simulink library "PC_Simulator_Lib"  (Simulink 8.2)
settings: Solver=ode45  StartTime=0.0  StopTime=10.0  RelTol=1e-3
values from neighbouring files (symbols this model uses):
  data = [r1 r2 r3 r4 L1 L2 L3 L4]    [strasse_Bedatung_HNI_ITI.m]
  distSameLane = 60    [InitialisationsEnv.m]
  eng_speed = [0 60 120 180 240 300 360 420 480 540 600 660 ... (101 elements, 1x101)]    [engine_table.mat]    (also in motor_parameter_calc.m = omega)
  Heading_init = 0    [Start.m]
  inertiaLateral = 25*(radiusWheel)^2    (= 4.129024)    [Start.m]
  laneWidth = 3.6    [InitialisationsEnv.m]    (also in strasse_Bedatung_HNI_ITI.m)
  omega_engine = [0.000000 150.000000 500.000000 1000.000000 1500.000000 2000.000000 2500.000000 3000.000000 3500.000000 4000.000000 4500.000000 5000.000000 5500.000000 6000.000000]    [friction_tables.m]
  omega_max = 6000    [engine_table.mat]    (also in motor_parameter_calc.m)
  omega_wheel = [0 20 40 60 80 100 122 143.7 164]    [friction_tables.m]
  para_Fellow_8_Points = ADAS.Fellow_8_Points    [ADAS_parameters.m]
  position_start_x = [x1 x2 x3 x4 x5 x6 x7]    [strasse_Bedatung_HNI_ITI.m]
  position_start_y = [y1 y2 y3 y4 y5 y6 y7]    [strasse_Bedatung_HNI_ITI.m]
  rad3rdLine = 57.2    [InitialisationsEnv.m]    (also in strasse_Bedatung_HNI_ITI.m)
  radiusWheel = 16*2.54/100    (= 0.4064)    [Start.m]
  s_values = [S1 S2 S3 S4 S5 S6 S7]    [strasse_Bedatung_HNI_ITI.m]
  segmentLimits = [segment1EndThirdLine                   segment2EndThirdLine                   segment3EndThirdLine                   segment4EndThirdLine                   segment5EndThirdLine                   segment6EndThirdLine                   segment7EndThirdLine                   segment8EndThirdLine                   ]    [InitialisationsEnv.m]    (also in strasse_Bedatung_HNI_ITI.m)
  setPosT = [-1.8 -5.4 -1.8 -5.4 -1.8 -5.4 -1.8 -5.4 -1.8 -5.4]    [InitialisationsEnv.m]
  torque = [297.089227105 300.997600937 304.800343044 308.497453426 312.088932082 315.574779014 318.95499422 322.229577701 325.398529457 328.461849487 331.419537793 334.271594373 ... (101 elements, 1x101)]    [engine_table.mat]    (also in motor_parameter_calc.m = g)
  Torque_lost = [0.000000 -8.777780 -15.000000 -26.800000 -29.600000 -32.700000 -35.900000 -39.300000 -42.800000 -46.500000 -50.300000 -54.300000 -58.500000 -62.800000 ]*0.6    [friction_tables.m]
  Torque_lost_wheel = [0.8 0.8 0.75 0.7 0.4 0.3 0.2 0.07 0.07]*0.2    [friction_tables.m]
  X_init = 0    [Start.m]
  Y_init = 1.8    [Start.m]
  Z_init = 0    [Start.m]
undefined symbols (not defined in the file or in its folder): Acc_Pedal, ADAS, Brake_Pedal, Joystick, Newton, Para, Raphson, Standard_Devices, Steering_Wheel_Angle, UDP_Protocol
libraries: simulink x43, rtwinlib x7, dspnetwork x2, simulink_extras x1, vrlib x1
(part 9 of 13)

== system PC_Simulator_Lib/Environment/Environment_Model/Traffic_Vehicle_Model1/Vehicle_Model_s ==
  note: Vehicle acceleration = 0.3 m/s2
  note: Actual S velocity [m/s]
  note: Desired S velocity [m/s]
  ResetSig[] : Inport
  VelSDesired[Km/h] : Inport  Port=2
  Integrate acceleration to speed : Integrator  ExternalReset=rising
  Integrate speed to position : Integrator  ExternalReset=rising  InitialCondition=Para.EN.InitCond.S01
  Proportional Gain : Gain  Gain=10
  "Reset s position " : Math  Operator=mod  SaturateOnIntegerOverflow=on
  Road max length[m] : Constant  Value=2159
  Sum : Sum  Inputs=|+-
  Traffic vehicle model s direction First order system : TransferFcn  Denominator=[1 2*pi/0.3 ]
  "Transforn from  Km/h to m/s " : Gain  Gain=1/3.6
  VelS[m/s] : Outport
  PosS[m] : Outport  Port=2
  wires:
  VelSDesired[Km/h]/1 -> "Transforn from  Km/h to m/s "/1
  Integrate speed to position/1 -> "Reset s position "/1
  Road max length[m]/1 -> "Reset s position "/2
  "Transforn from  Km/h to m/s "/1 -> Sum/1
  ResetSig[]/1 -> Integrate acceleration to speed/2, Integrate speed to position/2
  "Reset s position "/1 -> PosS[m]/1
  Traffic vehicle model s direction First order system/1 -> Integrate acceleration to speed/1
  Integrate acceleration to speed/1 -> Sum/2, Integrate speed to position/1, VelS[m/s]/1
  Proportional Gain/1 -> Traffic vehicle model s direction First order system/1
  Sum/1 -> Proportional Gain/1

== system PC_Simulator_Lib/Environment/Environment_Model/Traffic_Vehicle_Model11/Vehicle_Model_s ==
  note: Desired S velocity [m/s]
  note: Actual S velocity [m/s]
  note: Vehicle acceleration = 0.3 m/s2
  ResetSig[] : Inport
  VelSDesired[Km/h] : Inport  Port=2
  Integrate acceleration to speed : Integrator  ExternalReset=rising
  Integrate speed to position : Integrator  ExternalReset=rising  InitialCondition=Para.EN.InitCond.S10
  Proportional Gain : Gain  Gain=10
  "Reset s position " : Math  Operator=mod  SaturateOnIntegerOverflow=on
  Road max length[m] : Constant  Value=2159
  Sum : Sum  Inputs=|+-
  Traffic vehicle model s direction First order system : TransferFcn  Denominator=[1 2*pi/0.3 ]
  "Transforn from  Km/h to m/s " : Gain  Gain=1/3.6
  VelS[m/s] : Outport
  PosS[m] : Outport  Port=2
  wires:
  Proportional Gain/1 -> Traffic vehicle model s direction First order system/1
  Sum/1 -> Proportional Gain/1
  Integrate acceleration to speed/1 -> VelS[m/s]/1, Integrate speed to position/1, Sum/2
  Traffic vehicle model s direction First order system/1 -> Integrate acceleration to speed/1
  "Reset s position "/1 -> PosS[m]/1
  ResetSig[]/1 -> Integrate speed to position/2, Integrate acceleration to speed/2
  "Transforn from  Km/h to m/s "/1 -> Sum/1
  Road max length[m]/1 -> "Reset s position "/2
  Integrate speed to position/1 -> "Reset s position "/1
  VelSDesired[Km/h]/1 -> "Transforn from  Km/h to m/s "/1

== system PC_Simulator_Lib/Environment/Environment_Model/Traffic_Vehicle_Model11/Vehicle_Model_t ==
  ResetSig[] : Inport
  PosTDesired[m] : Inport  Port=2
  Controller : Subsystem
  Integrator : Integrator  ExternalReset=rising  InitialCondition=-9
  Simple_vehicle_model_lateral : TransferFcn  Denominator=[0.2 1]
  Sum : Sum  Inputs=|+-
  PosT[m] : Outport
  wires:
  Sum/1 -> Controller/2(t_diff)
  Controller/1(v_ref) -> Simple_vehicle_model_lateral/1
  Integrator/1 -> PosT[m]/1, Sum/2
  Simple_vehicle_model_lateral/1 -> Integrator/1
  PosTDesired[m]/1 -> Sum/1
  ResetSig[]/1 -> Controller/1(ResetSig[]), Integrator/2

== system PC_Simulator_Lib/Environment/Environment_Model/Traffic_Vehicle_Model2/Vehicle_Model_s ==
  note: Vehicle acceleration = 0.3 m/s2
  note: Actual S velocity [m/s]
  note: Desired S velocity [m/s]
  ResetSig[] : Inport
  VelSDesired[Km/h] : Inport  Port=2
  Integrate acceleration to speed : Integrator  ExternalReset=rising
  Integrate speed to position : Integrator  ExternalReset=rising  InitialCondition=Para.EN.InitCond.S02
  Proportional Gain : Gain  Gain=10
  "Reset s position " : Math  Operator=mod  SaturateOnIntegerOverflow=on
  Road max length[m] : Constant  Value=2159
  Sum : Sum  Inputs=|+-
  Traffic vehicle model s direction First order system : TransferFcn  Denominator=[1 2*pi/0.3 ]
  "Transforn from  Km/h to m/s " : Gain  Gain=1/3.6
  VelS[m/s] : Outport
  PosS[m] : Outport  Port=2
  wires:
  VelSDesired[Km/h]/1 -> "Transforn from  Km/h to m/s "/1
  Integrate speed to position/1 -> "Reset s position "/1
  Road max length[m]/1 -> "Reset s position "/2
  "Transforn from  Km/h to m/s "/1 -> Sum/1
  ResetSig[]/1 -> Integrate acceleration to speed/2, Integrate speed to position/2
  "Reset s position "/1 -> PosS[m]/1
  Traffic vehicle model s direction First order system/1 -> Integrate acceleration to speed/1
  Integrate acceleration to speed/1 -> Sum/2, Integrate speed to position/1, VelS[m/s]/1
  Proportional Gain/1 -> Traffic vehicle model s direction First order system/1
  Sum/1 -> Proportional Gain/1

== system PC_Simulator_Lib/Environment/Environment_Model/Traffic_Vehicle_Model3/Vehicle_Model_s ==
  note: Vehicle acceleration = 0.3 m/s2
  note: Actual S velocity [m/s]
  note: Desired S velocity [m/s]
  ResetSig[] : Inport
  VelSDesired[Km/h] : Inport  Port=2
  Integrate acceleration to speed : Integrator  ExternalReset=rising
  Integrate speed to position : Integrator  ExternalReset=rising  InitialCondition=Para.EN.InitCond.S03
  Proportional Gain : Gain  Gain=10
  "Reset s position " : Math  Operator=mod  SaturateOnIntegerOverflow=on
  Road max length[m] : Constant  Value=2159
  Sum : Sum  Inputs=|+-
  Traffic vehicle model s direction First order system : TransferFcn  Denominator=[1 2*pi/0.3 ]
  "Transforn from  Km/h to m/s " : Gain  Gain=1/3.6
  VelS[m/s] : Outport
  PosS[m] : Outport  Port=2
  wires:
  VelSDesired[Km/h]/1 -> "Transforn from  Km/h to m/s "/1
  Integrate speed to position/1 -> "Reset s position "/1
  Road max length[m]/1 -> "Reset s position "/2
  "Transforn from  Km/h to m/s "/1 -> Sum/1
  ResetSig[]/1 -> Integrate acceleration to speed/2, Integrate speed to position/2
  "Reset s position "/1 -> PosS[m]/1
  Traffic vehicle model s direction First order system/1 -> Integrate acceleration to speed/1
  Integrate acceleration to speed/1 -> Sum/2, Integrate speed to position/1, VelS[m/s]/1
  Proportional Gain/1 -> Traffic vehicle model s direction First order system/1
  Sum/1 -> Proportional Gain/1

== system PC_Simulator_Lib/Environment/Environment_Model/Traffic_Vehicle_Model4/Vehicle_Model_s ==
  note: Vehicle acceleration = 0.3 m/s2
  note: Actual S velocity [m/s]
  note: Desired S velocity [m/s]
  ResetSig[] : Inport
  VelSDesired[Km/h] : Inport  Port=2
  Integrate acceleration to speed : Integrator  ExternalReset=rising
  Integrate speed to position : Integrator  ExternalReset=rising  InitialCondition=Para.EN.InitCond.S04
  Proportional Gain : Gain  Gain=10
  "Reset s position " : Math  Operator=mod  SaturateOnIntegerOverflow=on
  Road max length[m] : Constant  Value=2159
  Sum : Sum  Inputs=|+-
  Traffic vehicle model s direction First order system : TransferFcn  Denominator=[1 2*pi/0.3 ]
  "Transforn from  Km/h to m/s " : Gain  Gain=1/3.6
  VelS[m/s] : Outport
  PosS[m] : Outport  Port=2
  wires:
  VelSDesired[Km/h]/1 -> "Transforn from  Km/h to m/s "/1
  Integrate speed to position/1 -> "Reset s position "/1
  Road max length[m]/1 -> "Reset s position "/2
  "Transforn from  Km/h to m/s "/1 -> Sum/1
  ResetSig[]/1 -> Integrate acceleration to speed/2, Integrate speed to position/2
  "Reset s position "/1 -> PosS[m]/1
  Traffic vehicle model s direction First order system/1 -> Integrate acceleration to speed/1
  Integrate acceleration to speed/1 -> Sum/2, Integrate speed to position/1, VelS[m/s]/1
  Proportional Gain/1 -> Traffic vehicle model s direction First order system/1
  Sum/1 -> Proportional Gain/1

== system PC_Simulator_Lib/Environment/Environment_Model/Traffic_Vehicle_Model5/Vehicle_Model_s ==
  note: Vehicle acceleration = 0.3 m/s2
  note: Actual S velocity [m/s]
  note: Desired S velocity [m/s]
  ResetSig[] : Inport
  VelSDesired[Km/h] : Inport  Port=2
  Integrate acceleration to speed : Integrator  ExternalReset=rising
  Integrate speed to position : Integrator  ExternalReset=rising  InitialCondition=Para.EN.InitCond.S05
  Proportional Gain : Gain  Gain=10
  "Reset s position " : Math  Operator=mod  SaturateOnIntegerOverflow=on
  Road max length[m] : Constant  Value=2159
  Sum : Sum  Inputs=|+-
  Traffic vehicle model s direction First order system : TransferFcn  Denominator=[1 2*pi/0.3 ]
  "Transforn from  Km/h to m/s " : Gain  Gain=1/3.6
  VelS[m/s] : Outport
  PosS[m] : Outport  Port=2
  wires:
  VelSDesired[Km/h]/1 -> "Transforn from  Km/h to m/s "/1
  Integrate speed to position/1 -> "Reset s position "/1
  Road max length[m]/1 -> "Reset s position "/2
  "Transforn from  Km/h to m/s "/1 -> Sum/1
  ResetSig[]/1 -> Integrate acceleration to speed/2, Integrate speed to position/2
  "Reset s position "/1 -> PosS[m]/1
  Traffic vehicle model s direction First order system/1 -> Integrate acceleration to speed/1
  Integrate acceleration to speed/1 -> Sum/2, Integrate speed to position/1, VelS[m/s]/1
  Proportional Gain/1 -> Traffic vehicle model s direction First order system/1
  Sum/1 -> Proportional Gain/1

== system PC_Simulator_Lib/Environment/Environment_Model/Traffic_Vehicle_Model6/Vehicle_Model_s ==
  note: Vehicle acceleration = 0.3 m/s2
  note: Actual S velocity [m/s]
  note: Desired S velocity [m/s]
  ResetSig[] : Inport
  VelSDesired[Km/h] : Inport  Port=2
  Integrate acceleration to speed : Integrator  ExternalReset=rising
  Integrate speed to position : Integrator  ExternalReset=rising  InitialCondition=Para.EN.InitCond.S06
  Proportional Gain : Gain  Gain=10
  "Reset s position " : Math  Operator=mod  SaturateOnIntegerOverflow=on
  Road max length[m] : Constant  Value=2159
  Sum : Sum  Inputs=|+-
  Traffic vehicle model s direction First order system : TransferFcn  Denominator=[1 2*pi/0.3 ]
  "Transforn from  Km/h to m/s " : Gain  Gain=1/3.6
  VelS[m/s] : Outport
  PosS[m] : Outport  Port=2
  wires:
  VelSDesired[Km/h]/1 -> "Transforn from  Km/h to m/s "/1
  Integrate speed to position/1 -> "Reset s position "/1
  Road max length[m]/1 -> "Reset s position "/2
  "Transforn from  Km/h to m/s "/1 -> Sum/1
  ResetSig[]/1 -> Integrate acceleration to speed/2, Integrate speed to position/2
  "Reset s position "/1 -> PosS[m]/1
  Traffic vehicle model s direction First order system/1 -> Integrate acceleration to speed/1
  Integrate acceleration to speed/1 -> Sum/2, Integrate speed to position/1, VelS[m/s]/1
  Proportional Gain/1 -> Traffic vehicle model s direction First order system/1
  Sum/1 -> Proportional Gain/1

== system PC_Simulator_Lib/Environment/Environment_Model/Traffic_Vehicle_Model7/Vehicle_Model_s ==
  note: Vehicle acceleration = 0.3 m/s2
  note: Actual S velocity [m/s]
  note: Desired S velocity [m/s]
  ResetSig[] : Inport
  VelSDesired[Km/h] : Inport  Port=2
  Integrate acceleration to speed : Integrator  ExternalReset=rising
  Integrate speed to position : Integrator  ExternalReset=rising  InitialCondition=Para.EN.InitCond.S07
  Proportional Gain : Gain  Gain=10
  "Reset s position " : Math  Operator=mod  SaturateOnIntegerOverflow=on
  Road max length[m] : Constant  Value=2159
  Sum : Sum  Inputs=|+-
  Traffic vehicle model s direction First order system : TransferFcn  Denominator=[1 2*pi/0.3 ]
  "Transforn from  Km/h to m/s " : Gain  Gain=1/3.6
  VelS[m/s] : Outport
  PosS[m] : Outport  Port=2
  wires:
  VelSDesired[Km/h]/1 -> "Transforn from  Km/h to m/s "/1
  Integrate speed to position/1 -> "Reset s position "/1
  Road max length[m]/1 -> "Reset s position "/2
  "Transforn from  Km/h to m/s "/1 -> Sum/1
  ResetSig[]/1 -> Integrate acceleration to speed/2, Integrate speed to position/2
  "Reset s position "/1 -> PosS[m]/1
  Traffic vehicle model s direction First order system/1 -> Integrate acceleration to speed/1
  Integrate acceleration to speed/1 -> Sum/2, Integrate speed to position/1, VelS[m/s]/1
  Proportional Gain/1 -> Traffic vehicle model s direction First order system/1
  Sum/1 -> Proportional Gain/1

== system PC_Simulator_Lib/Environment/Environment_Model/Traffic_Vehicle_Model8/Vehicle_Model_s ==
  note: Vehicle acceleration = 0.3 m/s2
  note: Actual S velocity [m/s]
  note: Desired S velocity [m/s]
  ResetSig[] : Inport
  VelSDesired[Km/h] : Inport  Port=2
  Integrate acceleration to speed : Integrator  ExternalReset=rising
  Integrate speed to position : Integrator  ExternalReset=rising  InitialCondition=Para.EN.InitCond.S08
  Proportional Gain : Gain  Gain=10
  "Reset s position " : Math  Operator=mod  SaturateOnIntegerOverflow=on
  Road max length[m] : Constant  Value=2159
  Sum : Sum  Inputs=|+-
  Traffic vehicle model s direction First order system : TransferFcn  Denominator=[1 2*pi/0.3 ]
  "Transforn from  Km/h to m/s " : Gain  Gain=1/3.6
  VelS[m/s] : Outport
  PosS[m] : Outport  Port=2
  wires:
  VelSDesired[Km/h]/1 -> "Transforn from  Km/h to m/s "/1
  Integrate speed to position/1 -> "Reset s position "/1
  Road max length[m]/1 -> "Reset s position "/2
  "Transforn from  Km/h to m/s "/1 -> Sum/1
  ResetSig[]/1 -> Integrate acceleration to speed/2, Integrate speed to position/2
  "Reset s position "/1 -> PosS[m]/1
  Traffic vehicle model s direction First order system/1 -> Integrate acceleration to speed/1
  Integrate acceleration to speed/1 -> Sum/2, Integrate speed to position/1, VelS[m/s]/1
  Proportional Gain/1 -> Traffic vehicle model s direction First order system/1
  Sum/1 -> Proportional Gain/1

== system PC_Simulator_Lib/Environment/Environment_Model/Traffic_Vehicle_Model9/Vehicle_Model_s ==
  note: Vehicle acceleration = 0.3 m/s2
  note: Actual S velocity [m/s]
  note: Desired S velocity [m/s]
  ResetSig[] : Inport
  VelSDesired[Km/h] : Inport  Port=2
  Integrate acceleration to speed : Integrator  ExternalReset=rising
  Integrate speed to position : Integrator  ExternalReset=rising  InitialCondition=Para.EN.InitCond.S09
  Proportional Gain : Gain  Gain=10
  "Reset s position " : Math  Operator=mod  SaturateOnIntegerOverflow=on
  Road max length[m] : Constant  Value=2159
  Sum : Sum  Inputs=|+-
  Traffic vehicle model s direction First order system : TransferFcn  Denominator=[1 2*pi/0.3 ]
  "Transforn from  Km/h to m/s " : Gain  Gain=1/3.6
  VelS[m/s] : Outport
  PosS[m] : Outport  Port=2
  wires:
  VelSDesired[Km/h]/1 -> "Transforn from  Km/h to m/s "/1
  Integrate speed to position/1 -> "Reset s position "/1
  Road max length[m]/1 -> "Reset s position "/2
  "Transforn from  Km/h to m/s "/1 -> Sum/1
  ResetSig[]/1 -> Integrate acceleration to speed/2, Integrate speed to position/2
  "Reset s position "/1 -> PosS[m]/1
  Traffic vehicle model s direction First order system/1 -> Integrate acceleration to speed/1
  Integrate acceleration to speed/1 -> Sum/2, Integrate speed to position/1, VelS[m/s]/1
  Proportional Gain/1 -> Traffic vehicle model s direction First order system/1
  Sum/1 -> Proportional Gain/1

== system PC_Simulator_Lib/Vehicle dynamics/Vertical_Dyn./suspention_System/Rear_Right_Suspention ==
  note: Fs=f0s+KU
  note: Fs=K(Lf-(L0 - U))
  note: U
  note: Spring_intial_length+Spring_precompressed_length = Spring_Free_length
  note: Vertical_Velocity_Z_vehicle_corner_RR
  Vertical_Displacement_Z_vehicle_corner_RR : Inport
  Vertical_Displacement_Z0 : Inport  Port=2
  intial_force_form_mass_rr : Inport  Port=3
  Add1 : Sum  Inputs=+++
  Add2 : Sum  Inputs=+-
  Constant : Constant  Value=0
  Constant2 : Constant  Value=Para.VD.Spring_intial_length.v
  Gain : Gain  Gain=Para.VD.Spring_Stifness_Rear.v
  Gain2 : Gain  Gain=Para.VD.Damper_Damping_Constant_Rear.v
  Relational Operator : RelationalOperator  Operator=>  OutDataTypeStr=boolean  ZeroCross=off
  Relational Operator1 : RelationalOperator  Operator=<  OutDataTypeStr=boolean  ZeroCross=off
  Saturation : Saturate  UpperLimit=Para.VD.Spring_intial_length.v-Para.VD.Spring_Lower_limit.v  LowerLimit=Para.VD.Spring_intial_length.v-Para.VD.Spring_Upper_limit.v
  Subtract : Sum  Inputs=+-
  Subtract1 : Sum  Inputs=+-
  Subtract2 : Sum  Inputs=+-
  Switch : Switch
  Switch1 : Switch
  Transfer Fcn : TransferFcn  Numerator=[1 0]  Denominator=[0.001 1]
  vertical_dynamics_tire : Subsystem
  Force_Suspention_RR : Outport
  Hight_Reer_Right : Outport  Port=2
  Z1 : Outport  Port=3
  Z2actual : Outport  Port=4
  wires:
  Subtract2/1 -> Hight_Reer_Right/1
  Constant2/1 -> Subtract2/1
  Transfer Fcn/1 -> Subtract1/2
  Vertical_Displacement_Z_vehicle_corner_RR/1 -> Subtract/2, Transfer Fcn/1, Switch/3
  Subtract/1 -> Saturation/1, Relational Operator/1, Relational Operator1/1
  Saturation/1 -> Gain/1, Subtract2/2, Add2/2, Relational Operator/2, Relational Operator1/2
  Add1/1 -> Force_Suspention_RR/1, vertical_dynamics_tire/1(Force_Suspention)
  Gain2/1 -> Add1/2
  Subtract1/1 -> Gain2/1
  Gain/1 -> Add1/1
  vertical_dynamics_tire/1(Vertical_Displacement_Z1_Wheel) -> Subtract/1, Z1/1, Add2/1
  Vertical_Displacement_Z0/1 -> vertical_dynamics_tire/2(Vertical_Displacement_Z0_Road)
  vertical_dynamics_tire/2(Vertical_Velocity_Z1_Wheel) -> Subtract1/1
  intial_force_form_mass_rr/1 -> vertical_dynamics_tire/3(intial_force_form_mass), Switch1/3
  Add2/1 -> Switch/1
  Relational Operator/1 -> Switch/2
  Switch/1 -> Z2actual/1
  Constant/1 -> Switch1/1
  Switch1/1 -> Add1/3
  Relational Operator1/1 -> Switch1/2

== system PC_Simulator_Lib/Vehicle dynamics/Vertical_Dyn./suspention_System/Rear_left_Suspention ==
  note: Vertical_Velocity_Z_vehicle_corner_RR
  note: Spring_intial_length+Spring_precompressed_length = Spring_Free_length
  note: U
  note: Fs=K(Lf-(L0 - U))
  note: Fs=f0s+KU
  Vertical_Displacement_Z_vehicle_corner_Rl : Inport
  Vertical_Displacement_Z0 : Inport  Port=2
  intial_force_form_mass_rl : Inport  Port=3
  Add1 : Sum  Inputs=+++
  Add2 : Sum  Inputs=+-
  Constant : Constant  Value=0
  Constant2 : Constant  Value=Para.VD.Spring_intial_length.v
  Gain : Gain  Gain=Para.VD.Spring_Stifness_Rear.v
  Gain2 : Gain  Gain=Para.VD.Damper_Damping_Constant_Rear.v
  Relational Operator : RelationalOperator  Operator=>  OutDataTypeStr=boolean  ZeroCross=off
  Relational Operator1 : RelationalOperator  Operator=<  OutDataTypeStr=boolean  ZeroCross=off
  Saturation : Saturate  UpperLimit=Para.VD.Spring_intial_length.v-Para.VD.Spring_Lower_limit.v  LowerLimit=Para.VD.Spring_intial_length.v-Para.VD.Spring_Upper_limit.v
  Subtract : Sum  Inputs=+-
  Subtract1 : Sum  Inputs=+-
  Subtract2 : Sum  Inputs=+-
  Switch : Switch
  Switch1 : Switch
  Transfer Fcn : TransferFcn  Numerator=[1 0]  Denominator=[0.001 1]
  vertical_dynamics_tire : Subsystem
  Force_Suspention_RL : Outport
  Hight_Reer_left : Outport  Port=2
  Z1 : Outport  Port=3
  Z2actual : Outport  Port=4
  wires:
  intial_force_form_mass_rl/1 -> vertical_dynamics_tire/3(intial_force_form_mass), Switch1/3
  vertical_dynamics_tire/2(Vertical_Velocity_Z1_Wheel) -> Subtract1/1
  Vertical_Displacement_Z0/1 -> vertical_dynamics_tire/2(Vertical_Displacement_Z0_Road)
  vertical_dynamics_tire/1(Vertical_Displacement_Z1_Wheel) -> Subtract/1, Z1/1, Add2/1
  Gain/1 -> Add1/1
  Subtract1/1 -> Gain2/1
  Gain2/1 -> Add1/2
  Add1/1 -> vertical_dynamics_tire/1(Force_Suspention), Force_Suspention_RL/1
  Saturation/1 -> Gain/1, Relational Operator/2, Subtract2/2, Add2/2, Relational Operator1/2
  Subtract/1 -> Saturation/1, Relational Operator/1, Relational Operator1/1
  Vertical_Displacement_Z_vehicle_corner_Rl/1 -> Switch/3, Transfer Fcn/1, Subtract/2
  Transfer Fcn/1 -> Subtract1/2
  Constant2/1 -> Subtract2/1
  Subtract2/1 -> Hight_Reer_left/1
  Add2/1 -> Switch/1
  Relational Operator/1 -> Switch/2
  Switch/1 -> Z2actual/1
  Constant/1 -> Switch1/1
  Switch1/1 -> Add1/3
  Relational Operator1/1 -> Switch1/2

== system PC_Simulator_Lib/Vehicle dynamics/Vertical_Dyn./suspention_System/front_left_Suspention ==
  note: Fs=f0s+KU
  note: Fs=K(Lf-(L0 - U))
  note: U
  note: Spring_intial_length+Spring_precompressed_length = Spring_Free_length
  note: Vertical_Velocity_Z_vehicle_corner_RR
  Vertical_Displacement_Z_vehicle_corner_fl : Inport
  Vertical_Displacement_Z0 : Inport  Port=2
  intial_force_form_mass_fl : Inport  Port=3
  Hight_front_right : Inport  Port=4
  Add1 : Sum  Inputs=++++
  Add2 : Sum  Inputs=+-
  Constant : Constant  Value=0
  Constant2 : Constant  Value=Para.VD.Spring_intial_length.v
  Gain : Gain  Gain=Para.VD.Spring_Stifness_Front.v
  Gain1 : Gain  Gain=Para.VD.AntiRoll_Stifness.v
  Gain2 : Gain  Gain=Para.VD.Damper_Damping_Constant_Front.v
  Relational Operator : RelationalOperator  Operator=>  OutDataTypeStr=boolean  ZeroCross=off
  Relational Operator1 : RelationalOperator  Operator=<  OutDataTypeStr=boolean  ZeroCross=off
  Saturation : Saturate  UpperLimit=Para.VD.Spring_intial_length.v-Para.VD.Spring_Lower_limit.v  LowerLimit=Para.VD.Spring_intial_length.v-Para.VD.Spring_Upper_limit.v  ZeroCross=off
  Subtract{,1..3} (4 alike) : Sum  Inputs=+-
  Switch : Switch
  Switch1 : Switch
  Transfer Fcn : TransferFcn  Numerator=[1 0]  Denominator=[0.001 1]
  vertical_dynamics_tire : Subsystem
  Force_Suspention_FL : Outport
  Hight_front_left : Outport  Port=2
  Z1 : Outport  Port=3
  Z2actual : Outport  Port=4
  wires:
  Subtract2/1 -> Hight_front_left/1, Subtract3/1
  Constant2/1 -> Subtract2/1
  Transfer Fcn/1 -> Subtract1/2
  Vertical_Displacement_Z_vehicle_corner_fl/1 -> Subtract/2, Transfer Fcn/1, Switch/3
  Subtract/1 -> Saturation/1, Relational Operator/1, Relational Operator1/1
  Saturation/1 -> Subtract2/2, Relational Operator/2, Add2/2, Relational Operator1/2, Gain/1
  Add1/1 -> vertical_dynamics_tire/1(Force_Suspention), Force_Suspention_FL/1
  Gain2/1 -> Add1/2
  Subtract1/1 -> Gain2/1
  Gain/1 -> Add1/1
  vertical_dynamics_tire/1(Vertical_Displacement_Z1_Wheel) -> Subtract/1, Z1/1, Add2/1
  Vertical_Displacement_Z0/1 -> vertical_dynamics_tire/2(Vertical_Displacement_Z0_Road)
  vertical_dynamics_tire/2(Vertical_Velocity_Z1_Wheel) -> Subtract1/1
  intial_force_form_mass_fl/1 -> vertical_dynamics_tire/3(intial_force_form_mass), Switch1/3
  Add2/1 -> Switch/1
  Relational Operator/1 -> Switch/2
  Switch/1 -> Z2actual/1
  Hight_front_right/1 -> Subtract3/2
  Subtract3/1 -> Gain1/1
  Gain1/1 -> Add1/4
  Constant/1 -> Switch1/1
  Switch1/1 -> Add1/3
  Relational Operator1/1 -> Switch1/2

== system PC_Simulator_Lib/Vehicle dynamics/Vertical_Dyn./suspention_System/front_right_Suspention ==
  note: Vertical_Velocity_Z_vehicle_corner_fr
  note: Spring_intial_length+Spring_precompressed_length = Spring_Free_length
  note: U
  note: Fs=K(Lf-(L0 - U))
  note: Fs=f0s+KU
  Vertical_Displacement_Z_vehicle_corner_fr : Inport
  Vertical_Displacement_Z0 : Inport  Port=2
  intial_force_form_mass_fr : Inport  Port=3
  Hight_front_left : Inport  Port=4
  Add1 : Sum  Inputs=++++
  Add2 : Sum  Inputs=+-
  Constant : Constant  Value=0
  Constant2 : Constant  Value=Para.VD.Spring_intial_length.v
  Gain : Gain  Gain=Para.VD.Spring_Stifness_Front.v
  Gain1 : Gain  Gain=Para.VD.AntiRoll_Stifness.v
  Gain2 : Gain  Gain=Para.VD.Damper_Damping_Constant_Front.v
  Relational Operator : RelationalOperator  Operator=>  OutDataTypeStr=boolean  ZeroCross=off
  Relational Operator1 : RelationalOperator  Operator=<  OutDataTypeStr=boolean  ZeroCross=off
  Saturation : Saturate  UpperLimit=Para.VD.Spring_intial_length.v-Para.VD.Spring_Lower_limit.v  LowerLimit=Para.VD.Spring_intial_length.v-Para.VD.Spring_Upper_limit.v
  Subtract{,1..3} (4 alike) : Sum  Inputs=+-
  Switch : Switch
  Switch1 : Switch
  Transfer Fcn : TransferFcn  Numerator=[1 0]  Denominator=[0.001 1]
  vertical_dynamics_tire : Subsystem
  Force_Suspention_FR : Outport
  Hight_front_right : Outport  Port=2
  Z1 : Outport  Port=3
  Z2actual : Outport  Port=4
  wires:
  intial_force_form_mass_fr/1 -> vertical_dynamics_tire/3(intial_force_form_mass), Switch1/3
  vertical_dynamics_tire/2(Vertical_Velocity_Z1_Wheel) -> Subtract1/1
  Vertical_Displacement_Z0/1 -> vertical_dynamics_tire/2(Vertical_Displacement_Z0_Road)
  vertical_dynamics_tire/1(Vertical_Displacement_Z1_Wheel) -> Subtract/1, Z1/1, Add2/1
  Gain/1 -> Add1/1
  Subtract1/1 -> Gain2/1
  Gain2/1 -> Add1/2
  Add1/1 -> vertical_dynamics_tire/1(Force_Suspention), Force_Suspention_FR/1
  Saturation/1 -> Gain/1, Subtract2/2, Relational Operator/2, Add2/2, Relational Operator1/2
  Subtract/1 -> Saturation/1, Relational Operator/1, Relational Operator1/1
  Vertical_Displacement_Z_vehicle_corner_fr/1 -> Subtract/2, Transfer Fcn/1, Switch/3
  Transfer Fcn/1 -> Subtract1/2
  Constant2/1 -> Subtract2/1
  Subtract2/1 -> Hight_front_right/1, Subtract3/1
  Add2/1 -> Switch/1
  Relational Operator/1 -> Switch/2
  Switch/1 -> Z2actual/1
  Gain1/1 -> Add1/4
  Subtract3/1 -> Gain1/1
  Hight_front_left/1 -> Subtract3/2
  Constant/1 -> Switch1/1
  Switch1/1 -> Add1/3
  Relational Operator1/1 -> Switch1/2

== system PC_Simulator_Lib/Vehicle dynamics/force_from_wheel_cordination_transformation/Steer_model/Force_Analysis ==
  note: FLysin
  note: FLxcos
  note: FLxsin
  note: FLycos
  note: FRxcos
  note: FRysin
  note: FRxsin
  note: FRycos
  note: + & -
  FL_Angle : Inport
  FR_Angle : Inport  Port=2
  FLx_T : Inport  Port=3
  FRx_T : Inport  Port=4
  FLy_T : Inport  Port=5
  FRy_T : Inport  Port=6
  ADD : Sum  Inputs=-+
  ADD1 : Sum
  ADD2 : Sum  Inputs=+-
  ADD3 : Sum
  Product{,1..7} (8 alike) : Product  RndMeth=Zero
  Trigonometric Function : Trigonometry  Operator=cos
  Trigonometric Function1 : Trigonometry
  Trigonometric Function2 : Trigonometry  Operator=cos
  Trigonometric Function3 : Trigonometry
  FLx : Outport
  FLy : Outport  Port=2
  FRx : Outport  Port=3
  FRy : Outport  Port=4
  wires:
  FL_Angle/1 -> Trigonometric Function/1, Trigonometric Function1/1
  FR_Angle/1 -> Trigonometric Function2/1, Trigonometric Function3/1
  Trigonometric Function/1 -> Product4/1, Product/1
  Product/1 -> ADD/2
  FLx_T/1 -> Product2/2, Product/2
  FLy_T/1 -> Product1/2, Product4/2
  Trigonometric Function1/1 -> Product1/1, Product2/1
  Product1/1 -> ADD/1
  Product2/1 -> ADD1/1
  Product4/1 -> ADD1/2
  FRx_T/1 -> Product3/1, Product6/1
  Trigonometric Function2/1 -> Product3/2, Product7/2
  Product3/1 -> ADD2/1
  FRy_T/1 -> Product5/2, Product7/1
  Product5/1 -> ADD2/2
  Product6/1 -> ADD3/1
  Product7/1 -> ADD3/2
  ADD/1 -> FLx/1
  ADD1/1 -> FLy/1
  ADD2/1 -> FRx/1
  ADD3/1 -> FRy/1
  Trigonometric Function3/1 -> Product5/1, Product6/2

== system PC_Simulator_Lib/Vehicle dynamics/force_from_wheel_cordination_transformation/Steer_model/Steer_Angel_Distribution1 ==
  note: Turning_Radius_Measured_From_The_Edge
  Steering_Angle_HMI_[-1 1] : Inport
  Divide : Product  Inputs=*/
  Divide1 : Product  Inputs=*/
  Divide2 : Product  Inputs=*/
  Gain1 : Gain  Gain=0.5
  Gain2 : Gain  Gain=2
  Minimum_Turning_Radius : Constant  Value=Para.VD.Minimum_Turning_Radius.v
  Sum : Sum  Inputs=|+-
  Sum1 : Sum  Inputs=|++
  Trigonometric Function : Trigonometry  Operator=atan
  Trigonometric Function1 : Trigonometry  Operator=atan
  Wheel_Base_Length : Constant  Value=Para.VD.Wheel_Base_Length.v
  Wheel_Base_Width : Constant  Value=Para.VD.Wheel_Base_Width.v
  FL_Angle : Outport
  FR_Angle : Outport  Port=2
  wires:
  Minimum_Turning_Radius/1 -> Divide/1
  Divide/1 -> Sum/1, Sum1/1
  Wheel_Base_Width/1 -> Gain1/1
  Wheel_Base_Length/1 -> Divide1/1, Divide2/1
  Divide1/1 -> Trigonometric Function/1
  Divide2/1 -> Trigonometric Function1/1
  Sum/1 -> Divide1/2
  Sum1/1 -> Divide2/2
  Gain1/1 -> Sum/2, Sum1/2
  Gain2/1 -> Divide/2
  Trigonometric Function/1 -> FL_Angle/1
  Trigonometric Function1/1 -> FR_Angle/1
  Steering_Angle_HMI_[-1 1]/1 -> Gain2/1

== system PC_Simulator_Lib/Vehicle dynamics/velocity/velocity_conditioning/Velocitytrim ==
  vin : Inport
  Abs : Abs
  Constant2 : Constant  Value=0
  Constant6 : Constant  Value=10*eps
  Relational Operator3 : RelationalOperator  Operator=>  OutDataTypeStr=boolean
  Switch4 : Switch
  vout : Outport
  wires:
  Abs/1 -> Relational Operator3/1
  Constant6/1 -> Relational Operator3/2
  Constant2/1 -> Switch4/3
  Relational Operator3/1 -> Switch4/2
  vin/1 -> Abs/1, Switch4/1
  Switch4/1 -> vout/1

== system PC_Simulator_Lib/Vehicle dynamics/velocity/velocity_conditioning/Velocitytrim1 ==
  vin : Inport
  Abs : Abs
  Constant2 : Constant  Value=0
  Constant6 : Constant  Value=10*eps
  Relational Operator3 : RelationalOperator  Operator=>  OutDataTypeStr=boolean
  Switch4 : Switch
  vout : Outport
  wires:
  Switch4/1 -> vout/1
  vin/1 -> Switch4/1, Abs/1
  Relational Operator3/1 -> Switch4/2
  Constant2/1 -> Switch4/3
  Constant6/1 -> Relational Operator3/2
  Abs/1 -> Relational Operator3/1

== system PC_Simulator_Lib/Vehicle dynamics/velocity/velocity_conditioning/Velocitytrim2 ==
  vin : Inport
  Abs : Abs
  Constant2 : Constant  Value=0
  Constant6 : Constant  Value=10*eps
  Relational Operator3 : RelationalOperator  Operator=>  OutDataTypeStr=boolean
  Switch4 : Switch
  vout : Outport
  wires:
  Abs/1 -> Relational Operator3/1
  Constant6/1 -> Relational Operator3/2
  Constant2/1 -> Switch4/3
  Relational Operator3/1 -> Switch4/2
  vin/1 -> Abs/1, Switch4/1
  Switch4/1 -> vout/1

== system PC_Simulator_Lib/Vehicle dynamics/velocity/velocity_conditioning/Velocitytrim3 ==
  vin : Inport
  Abs : Abs
  Constant2 : Constant  Value=0
  Constant6 : Constant  Value=10*eps
  Relational Operator3 : RelationalOperator  Operator=>  OutDataTypeStr=boolean
  Switch4 : Switch
  vout : Outport
  wires:
  Switch4/1 -> vout/1
  vin/1 -> Switch4/1, Abs/1
  Relational Operator3/1 -> Switch4/2
  Constant2/1 -> Switch4/3
  Constant6/1 -> Relational Operator3/2
  Abs/1 -> Relational Operator3/1

== system PC_Simulator_Lib/Vehicle dynamics/velocity/velocity_conditioning/Velocitytrim4 ==
  vin : Inport
  Abs : Abs
  Constant2 : Constant  Value=0
  Constant6 : Constant  Value=10*eps
  Relational Operator3 : RelationalOperator  Operator=>  OutDataTypeStr=boolean
  Switch4 : Switch
  vout : Outport
  wires:
  Switch4/1 -> vout/1
  vin/1 -> Switch4/1, Abs/1
  Relational Operator3/1 -> Switch4/2
  Constant2/1 -> Switch4/3
  Constant6/1 -> Relational Operator3/2
  Abs/1 -> Relational Operator3/1

== system PC_Simulator_Lib/Vehicle dynamics/velocity/velocity_conditioning/Velocitytrim5 ==
  vin : Inport
  Abs : Abs
  Constant2 : Constant  Value=0
  Constant6 : Constant  Value=10*eps
  Relational Operator3 : RelationalOperator  Operator=>  OutDataTypeStr=boolean
  Switch4 : Switch
  vout : Outport
  wires:
  Abs/1 -> Relational Operator3/1
  Constant6/1 -> Relational Operator3/2
  Constant2/1 -> Switch4/3
  Relational Operator3/1 -> Switch4/2
  vin/1 -> Abs/1, Switch4/1
  Switch4/1 -> vout/1

== system PC_Simulator_Lib/Vehicle dynamics/velocity/velocity_conditioning/Velocitytrim6 ==
  vin : Inport
  Abs : Abs
  Constant2 : Constant  Value=0
  Constant6 : Constant  Value=10*eps
  Relational Operator3 : RelationalOperator  Operator=>  OutDataTypeStr=boolean
  Switch4 : Switch
  vout : Outport
  wires:
  Switch4/1 -> vout/1
  vin/1 -> Switch4/1, Abs/1
  Relational Operator3/1 -> Switch4/2
  Constant2/1 -> Switch4/3
  Constant6/1 -> Relational Operator3/2
  Abs/1 -> Relational Operator3/1

== system PC_Simulator_Lib/Vehicle dynamics/velocity/velocity_conditioning/Velocitytrim7 ==
  vin : Inport
  Abs : Abs
  Constant2 : Constant  Value=0
  Constant6 : Constant  Value=10*eps
  Relational Operator3 : RelationalOperator  Operator=>  OutDataTypeStr=boolean
  Switch4 : Switch
  vout : Outport
  wires:
  Abs/1 -> Relational Operator3/1
  Constant6/1 -> Relational Operator3/2
  Constant2/1 -> Switch4/3
  Relational Operator3/1 -> Switch4/2
  vin/1 -> Abs/1, Switch4/1
  Switch4/1 -> vout/1

== system PC_Simulator_Lib/ADAS/Decision_Making_ADAS/Trajectory_calculatin_and_distance_control_and output_maping/Calculate_Desired_Trajectory/Curvature_Calculation ==
  Curvature_Road_Center[1|m] : Inport
  t_Value[m] : Inport  Port=2
  Constant : Constant
  Constant1 : Constant
  Divide : Product  Inputs=*/
  Divide1 : Product  Inputs=*/
  Subtract : Sum  Inputs=+-
  Curvature_Given_Point[1|m] : Outport
  wires:
  Constant/1 -> Divide/1
  Curvature_Road_Center[1|m]/1 -> Divide/2
  Divide/1 -> Subtract/1
  t_Value[m]/1 -> Subtract/2
  Constant1/1 -> Divide1/1
  Subtract/1 -> Divide1/2
  Divide1/1 -> Curvature_Given_Point[1|m]/1

== system PC_Simulator_Lib/ADAS/Decision_Making_ADAS/Trajectory_calculatin_and_distance_control_and output_maping/Calculate_Desired_Trajectory/Road model ST_XY ==
  note: Simple road model to transform the (s,t) point of the
      | local coordinate system to (x,y) point of the global
      | coordinate system
  note: Road model to transform
      | the (s,t) point to (x,y) point
  s[m] : Inport
  t[m] : Inport  Port=2
  Terminator1 : Terminator
  Terminator2 : Terminator
  Terminator3 : Terminator
  laneWidth : Constant  Value=laneWidth
  rad3rdLine : Constant  Value=rad3rdLine
  segmentLimits : Constant  Value=segmentLimits
  st_xy : MATLAB Function  TreatAsAtomicUnit=on
  x[m] : Outport
  y[m] : Outport  Port=2
  headingAngle[deg] : Outport  Port=3
  curvature[1/m] : Outport  Port=4
  wires:
  st_xy/7(segmentNr) -> Terminator2/1
  st_xy/6(friction) -> Terminator1/1
  st_xy/5(curvature) -> curvature[1/m]/1
  st_xy/4(headingAngle) -> headingAngle[deg]/1
  st_xy/3(z) -> Terminator3/1
  st_xy/2(y) -> y[m]/1
  st_xy/1(x) -> x[m]/1
  t[m]/1 -> st_xy/2(t)
  s[m]/1 -> st_xy/1(s)
  segmentLimits/1 -> st_xy/3(segmentLimits)
  laneWidth/1 -> st_xy/4(laneWidth)
  rad3rdLine/1 -> st_xy/5(rad3rdLine)

== system PC_Simulator_Lib/ADAS/Decision_Making_ADAS/Trajectory_calculatin_and_distance_control_and output_maping/Calculate_Desired_Trajectory/Strasse_xy ==
  x[m] : Inport
  y[m] : Inport  Port=2
  Constant : Constant  Value=data
  Constant1 : Constant  Value=position_start_x
  Constant2 : Constant  Value=position_start_y
  Constant3 : Constant  Value=s_values
  Embedded MATLAB Function : MATLAB Function  TreatAsAtomicUnit=on
  Terminator2 : Terminator
  Terminator3 : Terminator
  s[m] : Outport
  t[m] : Outport  Port=2
  Heading_angle[rad] : Outport  Port=3
  wires:
  Constant/1 -> Embedded MATLAB Function/1(data)
  Constant1/1 -> Embedded MATLAB Function/2(position_start_x)
  Constant2/1 -> Embedded MATLAB Function/3(position_start_y)
  Constant3/1 -> Embedded MATLAB Function/4(s_values)
  Embedded MATLAB Function/3(mue) -> Terminator2/1
  Embedded MATLAB Function/1(z) -> Terminator3/1
  x[m]/1 -> Embedded MATLAB Function/5(x)
  y[m]/1 -> Embedded MATLAB Function/6(y)
  Embedded MATLAB Function/4(s) -> s[m]/1
  Embedded MATLAB Function/5(t) -> t[m]/1
  Embedded MATLAB Function/2(psi) -> Heading_angle[rad]/1

== system PC_Simulator_Lib/ADAS/Decision_Making_ADAS/Trajectory_calculatin_and_distance_control_and output_maping/Calculate_Desired_Trajectory/adding_Delta_s_and_road_restart ==
  S_Virtual_Point_Actual[m] : Inport
  Vx_CoG[m|s] : Inport  Port=2
  Compare To Constant : simulink/Logic and Bit Operations/Compare To Constant  relop=>  const=segmentLimits(8)  OutDataTypeStr=boolean
  Compare To Constant1 : simulink/Logic and Bit Operations/Compare To Constant  relop=>  const=4  OutDataTypeStr=boolean
  Constant : Constant  Value=ADAS.Lateral_Control.delta_s
  Constant1 : Constant  Value=segmentLimits(8)
  Constant2 : Constant  Value=0
  Subtract : Sum  Inputs=+-
  Sum : Sum  Inputs=++|
  Switch : Switch  Criteria=u2 > Threshold
  Switch1 : Switch  Criteria=u2 > Threshold
  Terminator : Terminator
  S_Virtual_Point_Desired[m] : Outport
  wires:
  S_Virtual_Point_Actual[m]/1 -> Sum/2
  Compare To Constant/1 -> Switch/2
  Constant1/1 -> Subtract/2
  Subtract/1 -> Switch/1
  Switch/1 -> S_Virtual_Point_Desired[m]/1
  Sum/1 -> Switch/3, Subtract/1, Compare To Constant/1
  Vx_CoG[m|s]/1 -> Compare To Constant1/1
  Constant2/1 -> Switch1/3
  Compare To Constant1/1 -> Switch1/2
  Constant/1 -> Sum/1, Switch1/1
  Switch1/1 -> Terminator/1

== system PC_Simulator_Lib/ADAS/Decision_Making_ADAS/Trajectory_calculatin_and_distance_control_and output_maping/Calculate_Desired_Trajectory/applying_Desired_T_Gradually ==
  Enable_Lateral_Controller : Inport
  T_current[m] : Inport  Port=2
  T_Desired_initial[m] : Inport  Port=3
  Delta_T_Rate_limitl[m|s] : Inport  Port=4
  Vx_CoG[m|s] : Inport  Port=5
  Add : Sum  Inputs=-+
  Add1 : Sum
  Compare To Constant : simulink/Logic and Bit Operations/Compare To Constant  relop=>  const=0.2  OutDataTypeStr=boolean
  Data Type Conversion : DataTypeConversion
  Ground : Ground
  Memory : Memory
  Product : Product
  Product1 : Product
  Rate Limiter Dynamic : simulink/Discontinuities/Rate Limiter Dynamic
  Switch : Switch  Criteria=u2 > Threshold
  Terminator : Terminator
  Triggered Subsystem : Subsystem  TreatAsAtomicUnit=on
  Unary Minus : UnaryMinus
  T_Desired_execute[m] : Outport
  wires:
  Triggered Subsystem/1(Out1) -> Add1/1, Add/1
  T_Desired_initial[m]/1 -> Product/2
  Add/1 -> Rate Limiter Dynamic/2  "delta_t"
  Rate Limiter Dynamic/1 -> Add1/2
  Product/1 -> Add/2
  Data Type Conversion/1 -> Product1/2, Product/1
  Delta_T_Rate_limitl[m|s]/1 -> Rate Limiter Dynamic/1, Unary Minus/1
  Unary Minus/1 -> Rate Limiter Dynamic/3
  Product1/1 -> Triggered Subsystem/1(In1)
  Vx_CoG[m|s]/1 -> Compare To Constant/1
  Compare To Constant/1 -> Switch/2
  T_current[m]/1 -> Switch/3, Product1/1
  Enable_Lateral_Controller/1 -> Memory/1
  Add1/1 -> T_Desired_execute[m]/1
  Switch/1 -> Terminator/1
  Ground/1 -> Switch/1
  Memory/1 -> Data Type Conversion/1, Triggered Subsystem/Trigger

== system PC_Simulator_Lib/ADAS/Decision_Making_ADAS/Trajectory_calculatin_and_distance_control_and output_maping/Calculate_Desired_Trajectory/x_y_Virtual_Point_Calculation ==
  x[m] : Inport
  y[m] : Inport  Port=2
  Yaw_Angle[rad] : Inport  Port=3
  Add : Sum
  Add1 : Sum
  Distance_of_Virtual_Point : Constant  Value=ADAS.Lateral_Control.q
  Product : Product
  Product1 : Product
  Trigonometric Function : Trigonometry  Operator=cos
  Trigonometric Function1 : Trigonometry
  x_Virtual_Point[m] : Outport
  y_Virtual_Point[m] : Outport  Port=2
  wires:
  Yaw_Angle[rad]/1 -> Trigonometric Function1/1, Trigonometric Function/1
  Trigonometric Function/1 -> Product/2
  Trigonometric Function1/1 -> Product1/1
  Product/1 -> Add/2
  x[m]/1 -> Add/1
  Product1/1 -> Add1/1
  y[m]/1 -> Add1/2
  Distance_of_Virtual_Point/1 -> Product1/2, Product/1
  Add1/1 -> y_Virtual_Point[m]/1
  Add/1 -> x_Virtual_Point[m]/1

== system PC_Simulator_Lib/ADAS/Decision_Making_ADAS/Trajectory_calculatin_and_distance_control_and output_maping/Distance_Control/Calculate_distances ==
  acceleration_min[m|s2] : Inport
  V_realtive[m|s] : Inport  Port=2
  V_Vehicle[m|s] : Inport  Port=3
  Time_Gap_Desired[s] : Inport  Port=4
  Add : Sum
  Add1 : Sum
  Constant : Constant  Value=4
  Divide : Product  Inputs=*/
  Gain : Gain  Gain=-2
  Math Function : Math  Operator=square  SaturateOnIntegerOverflow=on
  Product : Product
  S_Start_Braking[m] : Outport
  Distance_Desired[m] : Outport  Port=2
  wires:
  V_realtive[m|s]/1 -> Math Function/1
  Math Function/1 -> Divide/1
  Gain/1 -> Divide/2
  acceleration_min[m|s2]/1 -> Gain/1
  Divide/1 -> Add/1  "Distance_Critical"
  V_Vehicle[m|s]/1 -> Product/1
  Time_Gap_Desired[s]/1 -> Product/2
  Product/1 -> Add1/1  "Distance_Desired"
  Add/1 -> S_Start_Braking[m]/1
  Constant/1 -> Add1/2
  Add1/1 -> Distance_Desired[m]/1, Add/2

== system PC_Simulator_Lib/ADAS/Decision_Making_ADAS/Trajectory_calculatin_and_distance_control_and output_maping/Distance_Control/Distance controller ==
  Distance_2_Felow_Vehicle[m] : Inport
  S_Start_Braking[m] : Inport  Port=2
  Distance_desired[m] : Inport  Port=3
  V_realtive[m|s] : Inport  Port=4
  V_Vehicle[m|s] : Inport  Port=5
  V_Desired_max[m|s] : Inport  Port=6
  V_Desired_min[m|s] : Inport  Port=7
  V_User_Set_Speed[m|s] : Inport  Port=8
  Control_law : Subsystem
  Enable_Distance_Controller : Subsystem
  Switch : Switch  Criteria=u2 > Threshold
  V_Desired_Following[m|s] : Outport
  wires:
  Control_law/1(V_Desired_Following[m|s]) -> Switch/1
  Distance_2_Felow_Vehicle[m]/1 -> Enable_Distance_Controller/2(Distance_2_Felow_Vehicle[m]), Control_law/2(Distance_acctual[m])
  V_Desired_max[m|s]/1 -> Control_law/5(V_Desired_max[m|s]), Switch/3
  Switch/1 -> V_Desired_Following[m|s]/1
  Distance_desired[m]/1 -> Control_law/1(Distance_desired[m])
  V_realtive[m|s]/1 -> Enable_Distance_Controller/3(V_realtive[m|s]), Control_law/3(V_realtive[m|s])
  V_Vehicle[m|s]/1 -> Enable_Distance_Controller/4(V_Vehicle[m|s]), Control_law/4(V_Vehicle[m|s])
  V_Desired_min[m|s]/1 -> Control_law/6(V_Desired_min[m|s])
  S_Start_Braking[m]/1 -> Enable_Distance_Controller/1(S_Start_Braking[m])
  Enable_Distance_Controller/1(Enable_Distance_Controller) -> Control_law/Enable, Switch/2
  V_User_Set_Speed[m|s]/1 -> Enable_Distance_Controller/5(V_User_Set_Speed[m|s])

== system PC_Simulator_Lib/ADAS/Execution_ADAS/Lateral_Controller_S_Function/Lateral_controller/Inverse_Steering_system ==
  Inner_Wheel_Steeringangle[rad] : Inport
  Abs : Abs
  Abs1 : Abs
  Add : Sum
  Add1 : Sum  Inputs=+-
  Divide3 : Product  Inputs=*/
  Divide4 : Product  Inputs=*/
  Divide6 : Product  Inputs=*/
  Gain3 : Gain  Gain=0.5
  Gain4 : Gain  Gain=0.5
  Gain6 : Gain  Gain=0.5
  Minimum_Turning_Radius1 : Constant  Value=Para.VD.Minimum_Turning_Radius.v
  Relational Operator : RelationalOperator  Operator=<  OutDataTypeStr=boolean
  Saturation : Saturate  UpperLimit=1  LowerLimit=-1
  Switch : Switch  Criteria=u2 > Threshold
  Trigonometric Function2 : Trigonometry  Operator=tan
  Wheel_Base_Length1 : Constant  Value=Para.VD.Wheel_Base_Length.v
  Wheel_Base_Width1 : Constant  Value=Para.VD.Wheel_Base_Width.v
  Steering_Wheel_Angle[norm] : Outport
  wires:
  Trigonometric Function2/1 -> Divide3/2
  Wheel_Base_Length1/1 -> Divide3/1
  Divide3/1 -> Add1/1, Add/1
  Wheel_Base_Width1/1 -> Gain3/1
  Gain3/1 -> Add1/2, Add/2
  Add/1 -> Divide4/2
  Minimum_Turning_Radius1/1 -> Divide6/1, Divide4/1
  Divide4/1 -> Gain4/1
  Inner_Wheel_Steeringangle[rad]/1 -> Trigonometric Function2/1
  Add1/1 -> Divide6/2
  Divide6/1 -> Gain6/1
  Abs/1 -> Relational Operator/1
  Abs1/1 -> Relational Operator/2
  Relational Operator/1 -> Switch/2
  Gain4/1 -> Switch/1, Abs/1
  Gain6/1 -> Switch/3, Abs1/1
  Switch/1 -> Saturation/1
  Saturation/1 -> Steering_Wheel_Angle[norm]/1

== system PC_Simulator_Lib/ADAS/Execution_ADAS/Lateral_Controller_S_Function/Lateral_controller/control_law ==
  x_CoG_Global : Inport
  y_CoG_Global : Inport  Port=2
  v_CoG : Inport  Port=3
  Slip_Angle : Inport  Port=4
  Yaw_Angle : Inport  Port=5
  Yaw_Rate : Inport  Port=6
  x_Desire : Inport  Port=7
  y_Desired : Inport  Port=8
  Yaw_Desired : Inport  Port=9
  Yaw_Rate_Desired : Inport  Port=10
  v_Desired : Inport  Port=11
  a_Desired : Inport  Port=12
  S-Function : S-Function  FunctionName=Lateral_Control  Parameters=ADAS.Lateral_Control.Damping,ADAS.Lateral_Control.time_constant,ADAS.Lateral_Control.q,Para.VD.Mass.v,Para.VD.Inertia_zz.v,Para.VD.Length_Front.v,Para.VD.Length_Rear.v,ADAS.Lateral_Control.C_av,ADAS.Lateral_Control.C_ah  EnableBusSupport=off
  Inner_Wheel_Steeringangle[rad] : Outport
  wires:
  Yaw_Rate/1 -> S-Function/6
  v_CoG/1 -> S-Function/3
  Yaw_Desired/1 -> S-Function/9
  Yaw_Angle/1 -> S-Function/5
  y_CoG_Global/1 -> S-Function/2
  x_Desire/1 -> S-Function/7
  y_Desired/1 -> S-Function/8
  v_Desired/1 -> S-Function/11
  Yaw_Rate_Desired/1 -> S-Function/10
  a_Desired/1 -> S-Function/12
  Slip_Angle/1 -> S-Function/4
  x_CoG_Global/1 -> S-Function/1
  S-Function/1 -> Inner_Wheel_Steeringangle[rad]/1

== system PC_Simulator_Lib/ADAS/Execution_ADAS/Longitudinal_Controller/Acceleration_Control/Brake_Pedal_Calculation ==
  Torque_Wheel_required[Nm] : Inport
  Omega_Engine[rad|s] : Inport  Port=2
  Gearbox_Gear_Ratio : Inport  Port=3
  Differential_Gear_Ratio : Inport  Port=4
  Abs : Abs
  Compare To Constant : simulink/Logic and Bit Operations/Compare To Constant  relop=<  const=5  OutDataTypeStr=boolean
  Compare To Constant1 : simulink/Logic and Bit Operations/Compare To Constant  relop=>=  const=5  OutDataTypeStr=boolean
  Data Type Conversion : DataTypeConversion
  Divide : Product  Inputs=*/*
  Gain1 : Gain  Gain=60/(2*pi)
  Product : Product  Inputs=3
  Saturation : Saturate  UpperLimit=0  LowerLimit=-inf
  Saturation1 : Saturate  UpperLimit=1  LowerLimit=0
  Subtract : Sum  Inputs=+-
  Torque_Brake_Max : Constant  Value=3*Para.DT.Torque_max_Brake.v
  frection : Lookup_n-D  NumberOfTableDimensions=1  BreakpointsForDimension1=omega_engine  BeginIndexSearchUsingPreviousIndexResult=on  Table=Torque_lost  InputSameDT=on
  Brake_Pedal[norm] : Outport
  Brake_control_is_inactive[bool] : Outport  Port=2
  wires:
  Torque_Wheel_required[Nm]/1 -> Subtract/1
  Gain1/1 -> frection/1
  frection/1 -> Product/1
  Omega_Engine[rad|s]/1 -> Gain1/1
  Subtract/1 -> Saturation/1
  Saturation/1 -> Abs/1
  Abs/1 -> Compare To Constant1/1, Compare To Constant/1, Divide/1
  Torque_Brake_Max/1 -> Divide/2
  Divide/1 -> Saturation1/1
  Saturation1/1 -> Brake_Pedal[norm]/1
  Gearbox_Gear_Ratio/1 -> Product/2
  Differential_Gear_Ratio/1 -> Product/3
  Product/1 -> Subtract/2
  Compare To Constant/1 -> Brake_control_is_inactive[bool]/1
  Compare To Constant1/1 -> Data Type Conversion/1
  Data Type Conversion/1 -> Divide/3

== system PC_Simulator_Lib/ADAS/Execution_ADAS/Longitudinal_Controller/Acceleration_Control/PI_Controller_plus_antiwindup_For_Brake ==
  a_desired[m|s2] : Inport
  a_acctual[m|s2] : Inport  Port=2
  Difference_on_sides_Saturation : Inport  Port=3
  Brake_control_is_inactive[bool] : Inport  Port=4
  Abs : Abs
  Add : Sum
  Compare To Zero : simulink/Logic and Bit Operations/Compare To Zero  relop=>  OutDataTypeStr=uint8
  Compare To Zero1 : simulink/Logic and Bit Operations/Compare To Zero  relop=<  OutDataTypeStr=uint8
  Constant : Constant  Value=0
  Data Type Conversion : DataTypeConversion
  Integrator : Integrator
  Ki : Gain  Gain=ADAS.Acceleration_Control.Brake_PI.Ki
  Kp : Gain  Gain=ADAS.Acceleration_Control.Brake_PI.Kp
  Logical Operator : Logic  AllPortsSameDT=off  OutDataTypeStr=boolean
  Logical Operator1 : Logic  Operator=NOT  AllPortsSameDT=off  OutDataTypeStr=boolean
  Product : Product  RndMeth=Zero
  Product1 : Product
  Product2 : Product
  Subtract1 : Sum  Inputs=+-
  Switch : Switch  Criteria=u2 > Threshold
  Brake_Pedal_Zusatz[norm] : Outport
  wires:
  Switch/1 -> Ki/1
  Logical Operator/1 -> Switch/2
  Brake_control_is_inactive[bool]/1 -> Logical Operator1/1
  Subtract1/1 -> Product1/1
  Compare To Zero1/1 -> Logical Operator/1
  Product/1 -> Compare To Zero1/1
  Difference_on_sides_Saturation/1 -> Abs/1
  Compare To Zero/1 -> Logical Operator/2
  Abs/1 -> Compare To Zero/1
  Kp/1 -> Add/1
  Integrator/1 -> Add/2
  Ki/1 -> Integrator/1
  Product1/1 -> Kp/1, Switch/3, Product/2
  a_acctual[m|s2]/1 -> Subtract1/2
  a_desired[m|s2]/1 -> Subtract1/1
  Add/1 -> Product/1, Product2/1
  Logical Operator1/1 -> Data Type Conversion/1
  Product2/1 -> Brake_Pedal_Zusatz[norm]/1
  Data Type Conversion/1 -> Product2/2, Product1/2
  Constant/1 -> Switch/1
